simulink model "LatticeFIR"  (R2020b)
settings: Solver=VariableStepAuto  StartTime=0.0  StopTime=40.0  RelTol=1e-3
undefined symbols (not defined in the file): b, K
libraries: dspsnks4 x1, dspvision x1
settings Model: Creator=Nic  LastModifiedBy=Nic

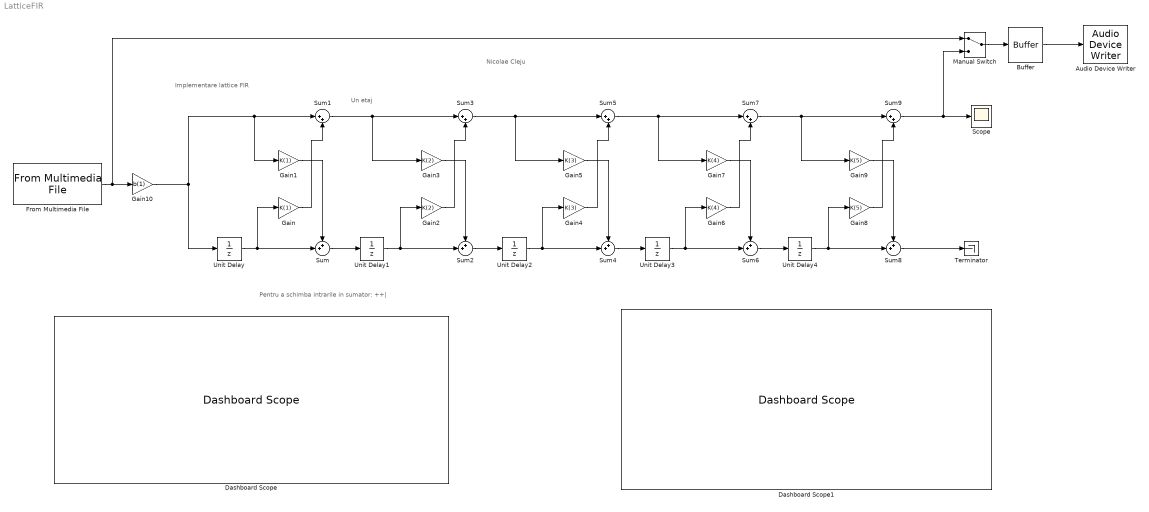
== system LatticeFIR ==
  note: Nicolae Cleju
  note: Implementare lattice FIR
  note: Un etaj
  note: Pentru a schimba intrarile in sumator: ++|
  Audio Device Writer : dspsnks4/Audio Device Writer  Driver=DirectSound  Device=Default  InheritSampleRate=on  SampleRate=44100  BitDepth=16-bit integer  BufferSize=4096  NumBuffers=10  DefaultOutputChannelMapping=on  OutputChannelMapping=1:2  OutputNumUnderrunSamples=off  DriverIdx=1  DeviceWarnFlag=''
  Buffer : Buffer  N=1024  OutputFrames=off
  Dashboard Scope : DashboardScope
  Dashboard Scope1 : DashboardScope
  From Multimedia File : dspvision/From Multimedia File  inputFilename=speech_dft.mp3  readRange=[1 Inf]  loop=on  numPlays=inf  outputStreams=Audio only  videoDataType=single  audioDataType=double  inheritSampleTime=on  userDefinedSampleTime=1/30  noAudioOutput=off  isIntensityVideo=off  fourcc=RGB  colorVideoFormat=Separate color signals  outputEOF=off  dataOrg=Column-major  audioFrameSize=1  computeAudioFrameSize=off  outSamplingMode=Sample based
  Gain : Gain  Gain=K(1)
  Gain1 : Gain  Gain=K(1)
  Gain10 : Gain  Gain=b(1)
  Gain2 : Gain  Gain=K(2)
  Gain3 : Gain  Gain=K(2)
  Gain4 : Gain  Gain=K(3)
  Gain5 : Gain  Gain=K(3)
  Gain6 : Gain  Gain=K(4)
  Gain7 : Gain  Gain=K(4)
  Gain8 : Gain  Gain=K(5)
  Gain9 : Gain  Gain=K(5)
  Manual Switch : ManualSwitch
  Scope : Scope
  Sum{,2,4,6,8} (5 alike) : Sum  Inputs=++|
  Sum{1,3,5,7,9} (5 alike) : Sum  Inputs=|++
  Terminator : Terminator
  Unit Delay{,1..4} (5 alike) : UnitDelay  SampleTime=-1  HasFrameUpgradeWarning=on
  wires:
  Unit Delay/1 -> Gain/1, Sum/2
  Gain/1 -> Sum1/2
  From Multimedia File/1 -> Manual Switch/1, Gain10/1
  Gain1/1 -> Sum/1
  Gain2/1 -> Sum3/2
  Unit Delay1/1 -> Gain2/1, Sum2/2
  Gain3/1 -> Sum2/1
  Sum1/1 -> Gain3/1, Sum3/1
  Sum/1 -> Unit Delay1/1
  Gain4/1 -> Sum5/2
  Unit Delay2/1 -> Gain4/1, Sum4/2
  Gain5/1 -> Sum4/1
  Sum3/1 -> Gain5/1, Sum5/1
  Sum2/1 -> Unit Delay2/1
  Gain6/1 -> Sum7/2
  Unit Delay3/1 -> Gain6/1, Sum6/2
  Gain7/1 -> Sum6/1
  Sum5/1 -> Gain7/1, Sum7/1
  Sum4/1 -> Unit Delay3/1
  Gain8/1 -> Sum9/2
  Unit Delay4/1 -> Gain8/1, Sum8/2
  Gain9/1 -> Sum8/1
  Sum9/1 -> Manual Switch/2, Scope/1
  Sum7/1 -> Gain9/1, Sum9/1
  Sum6/1 -> Unit Delay4/1
  Sum8/1 -> Terminator/1
  Buffer/1 -> Audio Device Writer/1
  Gain10/1 -> Gain1/1, Sum1/1, Unit Delay/1
  Manual Switch/1 -> Buffer/1
